simulink library "halout"  (R2021b)
settings: Solver=VariableStepAuto  StartTime=0.0  StopTime=10.0  RelTol=1e-3
undefined symbols (not defined in the file): C_TASK_5MS_S, FALSE, KHAL_CAN1TxReq_flg, KHAL_CAN2TxReq_flg, KHAL_CAN3FD3VCU1toNIDECTxReq_flg, KHAL_CAN3FD3VCU1TxReq_flg, KHAL_CAN3FD3VCU2E2E_flg, KHAL_CAN3FD3VCU2toNIDECE2E_flg, KHAL_CAN3FD3VCU2toNIDECTxReq_flg, KHAL_CAN3FD3VCU2TxReq_flg, KHAL_CAN3TxReq_flg, KHAL_CAN4FD4CE1000E2E_flg, KHAL_CAN4FD4CE1000TxReq_flg, KHAL_CAN4TxReq_flg, KHAL_CAN5TxReq_flg, KHAL_CAN7TxReq_flg, ONE_INT, TRUE, ZERO_INT
libraries: FVT_lib x258, simulink x115
(part 11 of 17)

== system halout/HAL_OUT/CAN2/FD2_CE200_1_0x435/FDCBCMKey2AccSta ==
  FDCBCMKey2AccSta : Inport
  Data Type Conversion : DataTypeConversion  OutDataTypeStr=uint8  RndMeth=Round
  CAN2_FDC_BCM_Key2Acc_Sta : Outport
  wires:
  Data Type Conversion/1 -> CAN2_FDC_BCM_Key2Acc_Sta/1
  FDCBCMKey2AccSta/1 -> Data Type Conversion/1

== system halout/HAL_OUT/CAN2/FD2_CE200_1_0x435/FDCBCMKey3AccSta ==
  FDCBCMKey3AccSta : Inport
  Data Type Conversion : DataTypeConversion  OutDataTypeStr=uint8  RndMeth=Round
  CAN2_FDC_BCM_Key3Acc_Sta : Outport
  wires:
  Data Type Conversion/1 -> CAN2_FDC_BCM_Key3Acc_Sta/1
  FDCBCMKey3AccSta/1 -> Data Type Conversion/1

== system halout/HAL_OUT/CAN2/FD2_CE200_1_0x435/FDCBCMKey4AccSta ==
  FDCBCMKey4AccSta : Inport
  Data Type Conversion : DataTypeConversion  OutDataTypeStr=uint8  RndMeth=Round
  CAN2_FDC_BCM_Key4Acc_Sta : Outport
  wires:
  Data Type Conversion/1 -> CAN2_FDC_BCM_Key4Acc_Sta/1
  FDCBCMKey4AccSta/1 -> Data Type Conversion/1

== system halout/HAL_OUT/CAN2/FD2_CE200_1_0x435/FDCBCMKey5AccSta ==
  FDCBCMKey5AccSta : Inport
  Data Type Conversion : DataTypeConversion  OutDataTypeStr=uint8  RndMeth=Round
  CAN2_FDC_BCM_Key5Acc_Sta : Outport
  wires:
  Data Type Conversion/1 -> CAN2_FDC_BCM_Key5Acc_Sta/1
  FDCBCMKey5AccSta/1 -> Data Type Conversion/1

== system halout/HAL_OUT/CAN2/FD2_CE200_1_0x435/FDCBCMKey6AccSta ==
  FDCBCMKey6AccSta : Inport
  Data Type Conversion : DataTypeConversion  OutDataTypeStr=uint8  RndMeth=Round
  CAN2_FDC_BCM_Key6Acc_Sta : Outport
  wires:
  Data Type Conversion/1 -> CAN2_FDC_BCM_Key6Acc_Sta/1
  FDCBCMKey6AccSta/1 -> Data Type Conversion/1

== system halout/HAL_OUT/CAN2/FD2_CE200_1_0x435/FDCBCMKey7AccSta ==
  FDCBCMKey7AccSta : Inport
  Data Type Conversion : DataTypeConversion  OutDataTypeStr=uint8  RndMeth=Round
  CAN2_FDC_BCM_Key7Acc_Sta : Outport
  wires:
  Data Type Conversion/1 -> CAN2_FDC_BCM_Key7Acc_Sta/1
  FDCBCMKey7AccSta/1 -> Data Type Conversion/1

== system halout/HAL_OUT/CAN2/FD2_CE200_1_0x435/FDCBCMKey8AccSta ==
  FDCBCMKey8AccSta : Inport
  Data Type Conversion : DataTypeConversion  OutDataTypeStr=uint8  RndMeth=Round
  CAN2_FDC_BCM_Key8Acc_Sta : Outport
  wires:
  Data Type Conversion/1 -> CAN2_FDC_BCM_Key8Acc_Sta/1
  FDCBCMKey8AccSta/1 -> Data Type Conversion/1

== system halout/HAL_OUT/CAN2/FD2_CE200_1_0x435/FDCBCMKey9AccSta ==
  FDCBCMKey9AccSta : Inport
  Data Type Conversion : DataTypeConversion  OutDataTypeStr=uint8  RndMeth=Round
  CAN2_FDC_BCM_Key9Acc_Sta : Outport
  wires:
  Data Type Conversion/1 -> CAN2_FDC_BCM_Key9Acc_Sta/1
  FDCBCMKey9AccSta/1 -> Data Type Conversion/1

== system halout/HAL_OUT/CAN2/FD2_CE200_1_0x435/FDCBCMLockAlarmCmd ==
  FDCBCMLockAlarmCmd : Inport
  Data Type Conversion : DataTypeConversion  OutDataTypeStr=uint8  RndMeth=Round
  CAN2_FDC_BCM_LockAlarm_Cmd : Outport
  wires:
  Data Type Conversion/1 -> CAN2_FDC_BCM_LockAlarm_Cmd/1
  FDCBCMLockAlarmCmd/1 -> Data Type Conversion/1

== system halout/HAL_OUT/CAN2/FD2_CE200_1_0x435/FDCBCMPTGOpenHeightSta ==
  FDCBCMPTGOpenHeightSta : Inport
  Data Type Conversion : DataTypeConversion  OutDataTypeStr=uint8  RndMeth=Round
  CAN2_FDC_BCM_PTGOpenHeight_Sta : Outport
  wires:
  Data Type Conversion/1 -> CAN2_FDC_BCM_PTGOpenHeight_Sta/1
  FDCBCMPTGOpenHeightSta/1 -> Data Type Conversion/1

== system halout/HAL_OUT/CAN2/FD2_CE200_1_0x435/FDCBCMRmLpModeENFunSta ==
  FDCBCMRmLpModeENFunSta : Inport
  Data Type Conversion : DataTypeConversion  OutDataTypeStr=uint8  RndMeth=Round
  CAN2_FDC_BCM_RmLpModeENFun_Sta : Outport
  wires:
  Data Type Conversion/1 -> CAN2_FDC_BCM_RmLpModeENFun_Sta/1
  FDCBCMRmLpModeENFunSta/1 -> Data Type Conversion/1

== system halout/HAL_OUT/CAN2/FD2_CE200_1_0x435/FDCBCMTurnSwTSetStaSta ==
  FDCBCMTurnSwTSetStaSta : Inport
  Data Type Conversion : DataTypeConversion  OutDataTypeStr=uint8  RndMeth=Round
  CAN2_FDC_BCM_TurnSwTSetSta_Sta : Outport
  wires:
  Data Type Conversion/1 -> CAN2_FDC_BCM_TurnSwTSetSta_Sta/1
  FDCBCMTurnSwTSetStaSta/1 -> Data Type Conversion/1

== system halout/HAL_OUT/CAN2/FD2_CE200_1_0x435/FDCBCMUserNowSta ==
  FDCBCMUserNowSta : Inport
  Data Type Conversion : DataTypeConversion  OutDataTypeStr=uint8  RndMeth=Round
  CAN2_FDC_BCM_UserNow_Sta : Outport
  wires:
  Data Type Conversion/1 -> CAN2_FDC_BCM_UserNow_Sta/1
  FDCBCMUserNowSta/1 -> Data Type Conversion/1

== system halout/HAL_OUT/CAN2/FD2_CE200_1_0x435/FDCBCMWalkInUnLkEnFunSta ==
  FDCBCMWalkInUnLkEnFunSta : Inport
  Data Type Conversion : DataTypeConversion  OutDataTypeStr=uint8  RndMeth=Round
  CAN2_FDC_BCM_WalkInUnLkEnFun_Sta : Outport
  wires:
  Data Type Conversion/1 -> CAN2_FDC_BCM_WalkInUnLkEnFun_Sta/1
  FDCBCMWalkInUnLkEnFunSta/1 -> Data Type Conversion/1

== system halout/HAL_OUT/CAN2/FD2_CE200_1_0x435/FDCBCMWalkOutLkEnFunSta ==
  FDCBCMWalkOutLkEnFunSta : Inport
  Data Type Conversion : DataTypeConversion  OutDataTypeStr=uint8  RndMeth=Round
  CAN2_FDC_BCM_WalkOutLkEnFun_Sta : Outport
  wires:
  Data Type Conversion/1 -> CAN2_FDC_BCM_WalkOutLkEnFun_Sta/1
  FDCBCMWalkOutLkEnFunSta/1 -> Data Type Conversion/1

== system halout/HAL_OUT/CAN2/FD2_CE200_1_0x435/FDCDKCDkeyShowIVISta ==
  FDCDKCDkeyShowIVISta : Inport
  Data Type Conversion : DataTypeConversion  OutDataTypeStr=uint8  RndMeth=Round
  CAN2_FDC_DKC_DkeyShowIVI_Sta : Outport
  wires:
  Data Type Conversion/1 -> CAN2_FDC_DKC_DkeyShowIVI_Sta/1
  FDCDKCDkeyShowIVISta/1 -> Data Type Conversion/1

== system halout/HAL_OUT/CAN2/FD2_CE200_1_0x435/FDCDKCKeyMissSta ==
  FDCDKCKeyMissSta : Inport
  Data Type Conversion : DataTypeConversion  OutDataTypeStr=uint8  RndMeth=Round
  CAN2_FDC_DKC_KeyMiss_Sta : Outport
  wires:
  Data Type Conversion/1 -> CAN2_FDC_DKC_KeyMiss_Sta/1
  FDCDKCKeyMissSta/1 -> Data Type Conversion/1

== system halout/HAL_OUT/CAN2/FD2_CE200_1_0x435/FDCDKCKeyNumSta ==
  FDCDKCKeyNumSta : Inport
  Data Type Conversion : DataTypeConversion  OutDataTypeStr=uint8  RndMeth=Round
  CAN2_FDC_DKC_KeyNum_Sta : Outport
  wires:
  Data Type Conversion/1 -> CAN2_FDC_DKC_KeyNum_Sta/1
  FDCDKCKeyNumSta/1 -> Data Type Conversion/1

== system halout/HAL_OUT/CAN2/FD2_CE200_1_0x435/FDCDKCKeyTypeSta ==
  FDCDKCKeyTypeSta : Inport
  Data Type Conversion : DataTypeConversion  OutDataTypeStr=uint8  RndMeth=Round
  CAN2_FDC_DKC_KeyType_Sta : Outport
  wires:
  Data Type Conversion/1 -> CAN2_FDC_DKC_KeyType_Sta/1
  FDCDKCKeyTypeSta/1 -> Data Type Conversion/1

== system halout/HAL_OUT/CAN2/FD2_CE200_1_0x435/FDCDKCUIDLowPowerSta ==
  FDCDKCUIDLowPowerSta : Inport
  Data Type Conversion : DataTypeConversion  OutDataTypeStr=uint8  RndMeth=Round
  CAN2_FDC_DKC_UIDLowPower_Sta : Outport
  wires:
  Data Type Conversion/1 -> CAN2_FDC_DKC_UIDLowPower_Sta/1
  FDCDKCUIDLowPowerSta/1 -> Data Type Conversion/1

== system halout/HAL_OUT/CAN2/FD2_CE200_1_0x435/FDCSPTGSPTGENFunSta ==
  FDCSPTGSPTGENFunSta : Inport
  Data Type Conversion : DataTypeConversion  OutDataTypeStr=uint8  RndMeth=Round
  CAN2_FDC_SPTG_SPTGENFun_Sta : Outport
  wires:
  Data Type Conversion/1 -> CAN2_FDC_SPTG_SPTGENFun_Sta/1
  FDCSPTGSPTGENFunSta/1 -> Data Type Conversion/1

== system halout/HAL_OUT/CAN2/FD2_CE200_1_0x435/FDCTHCMAPTCForceOFFSta ==
  FDCTHCMAPTCForceOFFSta : Inport
  Data Type Conversion : DataTypeConversion  OutDataTypeStr=uint8  RndMeth=Round
  CAN2_FDC_THCM_APTCForceOFF_Sta : Outport
  wires:
  Data Type Conversion/1 -> CAN2_FDC_THCM_APTCForceOFF_Sta/1
  FDCTHCMAPTCForceOFFSta/1 -> Data Type Conversion/1

== system halout/HAL_OUT/CAN2/FD2_CE200_1_0x435/FDCTHCMAPTCWarningSta ==
  FDCTHCMAPTCWarningSta : Inport
  Data Type Conversion : DataTypeConversion  OutDataTypeStr=uint8  RndMeth=Round
  CAN2_FDC_THCM_APTCWarning_Sta : Outport
  wires:
  Data Type Conversion/1 -> CAN2_FDC_THCM_APTCWarning_Sta/1
  FDCTHCMAPTCWarningSta/1 -> Data Type Conversion/1

== system halout/HAL_OUT/CAN2/FD2_CE200_1_0x435/FDCTHCMAirIntZ3Sta ==
  FDCTHCMAirIntZ3Sta : Inport
  Data Type Conversion : DataTypeConversion  OutDataTypeStr=uint8  RndMeth=Round
  CAN2_FDC_THCM_AirIntZ3_Sta : Outport
  wires:
  Data Type Conversion/1 -> CAN2_FDC_THCM_AirIntZ3_Sta/1
  FDCTHCMAirIntZ3Sta/1 -> Data Type Conversion/1

== system halout/HAL_OUT/CAN2/FD2_CE200_1_0x435/LFWheelShield ==
  LFWheelShield : Inport
  Data Type Conversion : DataTypeConversion  OutDataTypeStr=uint8  RndMeth=Round
  CAN2_LFWheelShield : Outport
  wires:
  Data Type Conversion/1 -> CAN2_LFWheelShield/1
  LFWheelShield/1 -> Data Type Conversion/1

== system halout/HAL_OUT/CAN2/FD2_CE200_1_0x435/LRBatWarn ==
  LRBatWarn : Inport
  Data Type Conversion : DataTypeConversion  OutDataTypeStr=uint8  RndMeth=Round
  CAN2_LRBatWarn : Outport
  wires:
  Data Type Conversion/1 -> CAN2_LRBatWarn/1
  LRBatWarn/1 -> Data Type Conversion/1

== system halout/HAL_OUT/CAN2/FD2_CE200_1_0x435/LRPressIndi ==
  LRPressIndi : Inport
  Data Type Conversion : DataTypeConversion  OutDataTypeStr=uint8  RndMeth=Round
  CAN2_LRPressIndi : Outport
  wires:
  Data Type Conversion/1 -> CAN2_LRPressIndi/1
  LRPressIndi/1 -> Data Type Conversion/1

== system halout/HAL_OUT/CAN2/FD2_CE200_1_0x435/LRSensorFail ==
  LRSensorFail : Inport
  Data Type Conversion : DataTypeConversion  OutDataTypeStr=uint8  RndMeth=Round
  CAN2_LRSensorFail : Outport
  wires:
  Data Type Conversion/1 -> CAN2_LRSensorFail/1
  LRSensorFail/1 -> Data Type Conversion/1

== system halout/HAL_OUT/CAN2/FD2_CE200_1_0x435/LRWheelDebug ==
  LRWheelDebug : Inport
  Data Type Conversion : DataTypeConversion  OutDataTypeStr=uint8  RndMeth=Round
  CAN2_LRWheelDebug : Outport
  wires:
  Data Type Conversion/1 -> CAN2_LRWheelDebug/1
  LRWheelDebug/1 -> Data Type Conversion/1

== system halout/HAL_OUT/CAN2/FD2_CE200_1_0x435/LRWheelPSW ==
  LRWheelPSW : Inport
  Data Type Conversion : DataTypeConversion  OutDataTypeStr=uint8  RndMeth=Round
  CAN2_LRWheelPSW : Outport
  wires:
  Data Type Conversion/1 -> CAN2_LRWheelPSW/1
  LRWheelPSW/1 -> Data Type Conversion/1

== system halout/HAL_OUT/CAN2/FD2_CE200_1_0x435/LRWheelPress ==
  LRWheelPress : Inport
  Data Type Conversion : DataTypeConversion  OutDataTypeStr=uint8  RndMeth=Round
  CAN2_LRWheelPress : Outport
  wires:
  Data Type Conversion/1 -> CAN2_LRWheelPress/1
  LRWheelPress/1 -> Data Type Conversion/1

== system halout/HAL_OUT/CAN2/FD2_CE200_1_0x435/LRWheelShield ==
  LRWheelShield : Inport
  Data Type Conversion : DataTypeConversion  OutDataTypeStr=uint8  RndMeth=Round
  CAN2_LRWheelShield : Outport
  wires:
  Data Type Conversion/1 -> CAN2_LRWheelShield/1
  LRWheelShield/1 -> Data Type Conversion/1

== system halout/HAL_OUT/CAN2/FD2_CE200_1_0x435/LRWheelTemp ==
  LRWheelTemp : Inport
  Data Type Conversion : DataTypeConversion  OutDataTypeStr=uint8  RndMeth=Round
  convert_out : FVT_lib/hal/convert_out  gain=1  offset=-40
  CAN2_LRWheelTemp : Outport
  wires:
  Data Type Conversion/1 -> CAN2_LRWheelTemp/1
  convert_out/1 -> Data Type Conversion/1
  LRWheelTemp/1 -> convert_out/1

== system halout/HAL_OUT/CAN2/FD2_CE200_1_0x435/LRWheelTmpIndi ==
  LRWheelTmpIndi : Inport
  Data Type Conversion : DataTypeConversion  OutDataTypeStr=uint8  RndMeth=Round
  CAN2_LRWheelTmpIndi : Outport
  wires:
  Data Type Conversion/1 -> CAN2_LRWheelTmpIndi/1
  LRWheelTmpIndi/1 -> Data Type Conversion/1

== system halout/HAL_OUT/CAN2/FD2_CE200_1_0x435/RFWheelShield ==
  RFWheelShield : Inport
  Data Type Conversion : DataTypeConversion  OutDataTypeStr=uint8  RndMeth=Round
  CAN2_RFWheelShield : Outport
  wires:
  Data Type Conversion/1 -> CAN2_RFWheelShield/1
  RFWheelShield/1 -> Data Type Conversion/1

== system halout/HAL_OUT/CAN2/FD2_CE200_1_0x435/RRBatWarn ==
  RRBatWarn : Inport
  Data Type Conversion : DataTypeConversion  OutDataTypeStr=uint8  RndMeth=Round
  CAN2_RRBatWarn : Outport
  wires:
  Data Type Conversion/1 -> CAN2_RRBatWarn/1
  RRBatWarn/1 -> Data Type Conversion/1

== system halout/HAL_OUT/CAN2/FD2_CE200_1_0x435/RRPressIndi ==
  RRPressIndi : Inport
  Data Type Conversion : DataTypeConversion  OutDataTypeStr=uint8  RndMeth=Round
  CAN2_RRPressIndi : Outport
  wires:
  Data Type Conversion/1 -> CAN2_RRPressIndi/1
  RRPressIndi/1 -> Data Type Conversion/1

== system halout/HAL_OUT/CAN2/FD2_CE200_1_0x435/RRSensorFail ==
  RRSensorFail : Inport
  Data Type Conversion : DataTypeConversion  OutDataTypeStr=uint8  RndMeth=Round
  CAN2_RRSensorFail : Outport
  wires:
  Data Type Conversion/1 -> CAN2_RRSensorFail/1
  RRSensorFail/1 -> Data Type Conversion/1

== system halout/HAL_OUT/CAN2/FD2_CE200_1_0x435/RRWheelDebug ==
  RRWheelDebug : Inport
  Data Type Conversion : DataTypeConversion  OutDataTypeStr=uint8  RndMeth=Round
  CAN2_RRWheelDebug : Outport
  wires:
  Data Type Conversion/1 -> CAN2_RRWheelDebug/1
  RRWheelDebug/1 -> Data Type Conversion/1

== system halout/HAL_OUT/CAN2/FD2_CE200_1_0x435/RRWheelPSW ==
  RRWheelPSW : Inport
  Data Type Conversion : DataTypeConversion  OutDataTypeStr=uint8  RndMeth=Round
  CAN2_RRWheelPSW : Outport
  wires:
  Data Type Conversion/1 -> CAN2_RRWheelPSW/1
  RRWheelPSW/1 -> Data Type Conversion/1

== system halout/HAL_OUT/CAN2/FD2_CE200_1_0x435/RRWheelPress ==
  RRWheelPress : Inport
  Data Type Conversion : DataTypeConversion  OutDataTypeStr=uint8  RndMeth=Round
  CAN2_RRWheelPress : Outport
  wires:
  Data Type Conversion/1 -> CAN2_RRWheelPress/1
  RRWheelPress/1 -> Data Type Conversion/1

== system halout/HAL_OUT/CAN2/FD2_CE200_1_0x435/RRWheelShield ==
  RRWheelShield : Inport
  Data Type Conversion : DataTypeConversion  OutDataTypeStr=uint8  RndMeth=Round
  CAN2_RRWheelShield : Outport
  wires:
  Data Type Conversion/1 -> CAN2_RRWheelShield/1
  RRWheelShield/1 -> Data Type Conversion/1

== system halout/HAL_OUT/CAN2/FD2_CE200_1_0x435/RRWheelTemp ==
  RRWheelTemp : Inport
  Data Type Conversion : DataTypeConversion  OutDataTypeStr=uint8  RndMeth=Round
  convert_out : FVT_lib/hal/convert_out  gain=1  offset=-40
  CAN2_RRWheelTemp : Outport
  wires:
  Data Type Conversion/1 -> CAN2_RRWheelTemp/1
  convert_out/1 -> Data Type Conversion/1
  RRWheelTemp/1 -> convert_out/1

== system halout/HAL_OUT/CAN2/FD2_CE200_1_0x435/RRWheelTmpIndi ==
  RRWheelTmpIndi : Inport
  Data Type Conversion : DataTypeConversion  OutDataTypeStr=uint8  RndMeth=Round
  CAN2_RRWheelTmpIndi : Outport
  wires:
  Data Type Conversion/1 -> CAN2_RRWheelTmpIndi/1
  RRWheelTmpIndi/1 -> Data Type Conversion/1

== system halout/HAL_OUT/CAN2/FD2_CE200_1_0x435/T1TPMSLFBatWarn ==
  T1TPMSLFBatWarn : Inport
  Data Type Conversion : DataTypeConversion  OutDataTypeStr=uint8  RndMeth=Round
  CAN2_T1_TPMS_LFBatWarn : Outport
  wires:
  Data Type Conversion/1 -> CAN2_T1_TPMS_LFBatWarn/1
  T1TPMSLFBatWarn/1 -> Data Type Conversion/1

== system halout/HAL_OUT/CAN2/FD2_CE200_1_0x435/T1TPMSLFPressIndi ==
  T1TPMSLFPressIndi : Inport
  Data Type Conversion : DataTypeConversion  OutDataTypeStr=uint8  RndMeth=Round
  CAN2_T1_TPMS_LFPressIndi : Outport
  wires:
  Data Type Conversion/1 -> CAN2_T1_TPMS_LFPressIndi/1
  T1TPMSLFPressIndi/1 -> Data Type Conversion/1

== system halout/HAL_OUT/CAN2/FD2_CE200_1_0x435/T1TPMSLFSensorFail ==
  T1TPMSLFSensorFail : Inport
  Data Type Conversion : DataTypeConversion  OutDataTypeStr=uint8  RndMeth=Round
  CAN2_T1_TPMS_LFSensorFail : Outport
  wires:
  Data Type Conversion/1 -> CAN2_T1_TPMS_LFSensorFail/1
  T1TPMSLFSensorFail/1 -> Data Type Conversion/1

== system halout/HAL_OUT/CAN2/FD2_CE200_1_0x435/T1TPMSLFWheelDebug ==
  T1TPMSLFWheelDebug : Inport
  Data Type Conversion : DataTypeConversion  OutDataTypeStr=uint8  RndMeth=Round
  CAN2_T1_TPMS_LFWheelDebug : Outport
  wires:
  Data Type Conversion/1 -> CAN2_T1_TPMS_LFWheelDebug/1
  T1TPMSLFWheelDebug/1 -> Data Type Conversion/1

== system halout/HAL_OUT/CAN2/FD2_CE200_1_0x435/T1TPMSLFWheelPSW ==
  T1TPMSLFWheelPSW : Inport
  Data Type Conversion : DataTypeConversion  OutDataTypeStr=uint8  RndMeth=Round
  CAN2_T1_TPMS_LFWheelPSW : Outport
  wires:
  Data Type Conversion/1 -> CAN2_T1_TPMS_LFWheelPSW/1
  T1TPMSLFWheelPSW/1 -> Data Type Conversion/1

== system halout/HAL_OUT/CAN2/FD2_CE200_1_0x435/T1TPMSLFWheelPress ==
  T1TPMSLFWheelPress : Inport
  Data Type Conversion : DataTypeConversion  OutDataTypeStr=uint8  RndMeth=Round
  CAN2_T1_TPMS_LFWheelPress : Outport
  wires:
  Data Type Conversion/1 -> CAN2_T1_TPMS_LFWheelPress/1
  T1TPMSLFWheelPress/1 -> Data Type Conversion/1

== system halout/HAL_OUT/CAN2/FD2_CE200_1_0x435/T1TPMSLFWheelTemp ==
  T1TPMSLFWheelTemp : Inport
  Data Type Conversion : DataTypeConversion  OutDataTypeStr=uint8  RndMeth=Round
  convert_out : FVT_lib/hal/convert_out  gain=1  offset=-40
  CAN2_T1_TPMS_LFWheelTemp : Outport
  wires:
  Data Type Conversion/1 -> CAN2_T1_TPMS_LFWheelTemp/1
  convert_out/1 -> Data Type Conversion/1
  T1TPMSLFWheelTemp/1 -> convert_out/1

== system halout/HAL_OUT/CAN2/FD2_CE200_1_0x435/T1TPMSLFWheelTmpIndi ==
  T1TPMSLFWheelTmpIndi : Inport
  Data Type Conversion : DataTypeConversion  OutDataTypeStr=uint8  RndMeth=Round
  CAN2_T1_TPMS_LFWheelTmpIndi : Outport
  wires:
  Data Type Conversion/1 -> CAN2_T1_TPMS_LFWheelTmpIndi/1
  T1TPMSLFWheelTmpIndi/1 -> Data Type Conversion/1

== system halout/HAL_OUT/CAN2/FD2_CE200_1_0x435/T1TPMSRFBatWarn ==
  T1TPMSRFBatWarn : Inport
  Data Type Conversion : DataTypeConversion  OutDataTypeStr=uint8  RndMeth=Round
  CAN2_T1_TPMS_RFBatWarn : Outport
  wires:
  Data Type Conversion/1 -> CAN2_T1_TPMS_RFBatWarn/1
  T1TPMSRFBatWarn/1 -> Data Type Conversion/1

== system halout/HAL_OUT/CAN2/FD2_CE200_1_0x435/T1TPMSRFPressIndi ==
  T1TPMSRFPressIndi : Inport
  Data Type Conversion : DataTypeConversion  OutDataTypeStr=uint8  RndMeth=Round
  CAN2_T1_TPMS_RFPressIndi : Outport
  wires:
  Data Type Conversion/1 -> CAN2_T1_TPMS_RFPressIndi/1
  T1TPMSRFPressIndi/1 -> Data Type Conversion/1

== system halout/HAL_OUT/CAN2/FD2_CE200_1_0x435/T1TPMSRFSensorFail ==
  T1TPMSRFSensorFail : Inport
  Data Type Conversion : DataTypeConversion  OutDataTypeStr=uint8  RndMeth=Round
  CAN2_T1_TPMS_RFSensorFail : Outport
  wires:
  Data Type Conversion/1 -> CAN2_T1_TPMS_RFSensorFail/1
  T1TPMSRFSensorFail/1 -> Data Type Conversion/1

== system halout/HAL_OUT/CAN2/FD2_CE200_1_0x435/T1TPMSRFWheelDebug ==
  T1TPMSRFWheelDebug : Inport
  Data Type Conversion : DataTypeConversion  OutDataTypeStr=uint8  RndMeth=Round
  CAN2_T1_TPMS_RFWheelDebug : Outport
  wires:
  Data Type Conversion/1 -> CAN2_T1_TPMS_RFWheelDebug/1
  T1TPMSRFWheelDebug/1 -> Data Type Conversion/1

== system halout/HAL_OUT/CAN2/FD2_CE200_1_0x435/T1TPMSRFWheelPSW ==
  T1TPMSRFWheelPSW : Inport
  Data Type Conversion : DataTypeConversion  OutDataTypeStr=uint8  RndMeth=Round
  CAN2_T1_TPMS_RFWheelPSW : Outport
  wires:
  Data Type Conversion/1 -> CAN2_T1_TPMS_RFWheelPSW/1
  T1TPMSRFWheelPSW/1 -> Data Type Conversion/1

== system halout/HAL_OUT/CAN2/FD2_CE200_1_0x435/T1TPMSRFWheelPress ==
  T1TPMSRFWheelPress : Inport
  Data Type Conversion : DataTypeConversion  OutDataTypeStr=uint8  RndMeth=Round
  CAN2_T1_TPMS_RFWheelPress : Outport
  wires:
  Data Type Conversion/1 -> CAN2_T1_TPMS_RFWheelPress/1
  T1TPMSRFWheelPress/1 -> Data Type Conversion/1

== system halout/HAL_OUT/CAN2/FD2_CE200_1_0x435/T1TPMSRFWheelTemp ==
  T1TPMSRFWheelTemp : Inport
  Data Type Conversion : DataTypeConversion  OutDataTypeStr=uint8  RndMeth=Round
  convert_out : FVT_lib/hal/convert_out  gain=1  offset=-40
  CAN2_T1_TPMS_RFWheelTemp : Outport
  wires:
  Data Type Conversion/1 -> CAN2_T1_TPMS_RFWheelTemp/1
  convert_out/1 -> Data Type Conversion/1
  T1TPMSRFWheelTemp/1 -> convert_out/1

== system halout/HAL_OUT/CAN2/FD2_CE200_1_0x435/T1TPMSRFWheelTmpIndi ==
  T1TPMSRFWheelTmpIndi : Inport
  Data Type Conversion : DataTypeConversion  OutDataTypeStr=uint8  RndMeth=Round
  CAN2_T1_TPMS_RFWheelTmpIndi : Outport
  wires:
  Data Type Conversion/1 -> CAN2_T1_TPMS_RFWheelTmpIndi/1
  T1TPMSRFWheelTmpIndi/1 -> Data Type Conversion/1

== system halout/HAL_OUT/CAN2/FD2_CE200_1_0x435/T1TPMSTPMSWarnIndi ==
  T1TPMSTPMSWarnIndi : Inport
  Data Type Conversion : DataTypeConversion  OutDataTypeStr=uint8  RndMeth=Round
  CAN2_T1_TPMS_TPMSWarnIndi : Outport
  wires:
  Data Type Conversion/1 -> CAN2_T1_TPMS_TPMSWarnIndi/1
  T1TPMSTPMSWarnIndi/1 -> Data Type Conversion/1

== system halout/HAL_OUT/CAN2/FD2_CE200_1_0x435/TPMSCaliButtAllow ==
  TPMSCaliButtAllow : Inport
  Data Type Conversion : DataTypeConversion  OutDataTypeStr=uint8  RndMeth=Round
  CAN2_TPMS_Cali_Butt_Allow : Outport
  wires:
  Data Type Conversion/1 -> CAN2_TPMS_Cali_Butt_Allow/1
  TPMSCaliButtAllow/1 -> Data Type Conversion/1

== system halout/HAL_OUT/CAN2/FD2_CE200_1_0x435/TPMSResButtAllow ==
  TPMSResButtAllow : Inport
  Data Type Conversion : DataTypeConversion  OutDataTypeStr=uint8  RndMeth=Round
  CAN2_TPMS_Res_Butt_Allow : Outport
  wires:
  Data Type Conversion/1 -> CAN2_TPMS_Res_Butt_Allow/1
  TPMSResButtAllow/1 -> Data Type Conversion/1

== system halout/HAL_OUT/CAN2/FD2_Version_0x3C3/FUSIONHWVer1 ==
  FUSIONHWVer1 : Inport
  Data Type Conversion : DataTypeConversion  OutDataTypeStr=uint8  RndMeth=Round
  CAN2_FUSION_HW_Ver1 : Outport
  wires:
  Data Type Conversion/1 -> CAN2_FUSION_HW_Ver1/1
  FUSIONHWVer1/1 -> Data Type Conversion/1

== system halout/HAL_OUT/CAN2/FD2_Version_0x3C3/FUSIONHWVer2 ==
  FUSIONHWVer2 : Inport
  Data Type Conversion : DataTypeConversion  OutDataTypeStr=uint8  RndMeth=Round
  CAN2_FUSION_HW_Ver2 : Outport
  wires:
  Data Type Conversion/1 -> CAN2_FUSION_HW_Ver2/1
  FUSIONHWVer2/1 -> Data Type Conversion/1

== system halout/HAL_OUT/CAN2/FD2_Version_0x3C3/FUSIONHWVer3 ==
  FUSIONHWVer3 : Inport
  Data Type Conversion : DataTypeConversion  OutDataTypeStr=uint8  RndMeth=Round
  CAN2_FUSION_HW_Ver3 : Outport
  wires:
  Data Type Conversion/1 -> CAN2_FUSION_HW_Ver3/1
  FUSIONHWVer3/1 -> Data Type Conversion/1

== system halout/HAL_OUT/CAN2/FD2_Version_0x3C3/FUSIONSWCarModel1 ==
  FUSIONSWCarModel1 : Inport
  Data Type Conversion : DataTypeConversion  OutDataTypeStr=uint8  RndMeth=Round
  CAN2_FUSION_SW_CarModel1 : Outport
  wires:
  Data Type Conversion/1 -> CAN2_FUSION_SW_CarModel1/1
  FUSIONSWCarModel1/1 -> Data Type Conversion/1

== system halout/HAL_OUT/CAN2/FD2_Version_0x3C3/FUSIONSWCarModel2 ==
  FUSIONSWCarModel2 : Inport
  Data Type Conversion : DataTypeConversion  OutDataTypeStr=uint8  RndMeth=Round
  CAN2_FUSION_SW_CarModel2 : Outport
  wires:
  Data Type Conversion/1 -> CAN2_FUSION_SW_CarModel2/1
  FUSIONSWCarModel2/1 -> Data Type Conversion/1

== system halout/HAL_OUT/CAN2/FD2_Version_0x3C3/FUSIONSWCarModel3 ==
  FUSIONSWCarModel3 : Inport
  Data Type Conversion : DataTypeConversion  OutDataTypeStr=uint8  RndMeth=Round
  CAN2_FUSION_SW_CarModel3 : Outport
  wires:
  Data Type Conversion/1 -> CAN2_FUSION_SW_CarModel3/1
  FUSIONSWCarModel3/1 -> Data Type Conversion/1

== system halout/HAL_OUT/CAN2/FD2_Version_0x3C3/FUSIONSWController1 ==
  FUSIONSWController1 : Inport
  Data Type Conversion : DataTypeConversion  OutDataTypeStr=uint8  RndMeth=Round
  CAN2_FUSION_SW_Controller1 : Outport
  wires:
  Data Type Conversion/1 -> CAN2_FUSION_SW_Controller1/1
  FUSIONSWController1/1 -> Data Type Conversion/1

== system halout/HAL_OUT/CAN2/FD2_Version_0x3C3/FUSIONSWController2 ==
  FUSIONSWController2 : Inport
  Data Type Conversion : DataTypeConversion  OutDataTypeStr=uint8  RndMeth=Round
  CAN2_FUSION_SW_Controller2 : Outport
  wires:
  Data Type Conversion/1 -> CAN2_FUSION_SW_Controller2/1
  FUSIONSWController2/1 -> Data Type Conversion/1

== system halout/HAL_OUT/CAN2/FD2_Version_0x3C3/FUSIONSWCountry1 ==
  FUSIONSWCountry1 : Inport
  Data Type Conversion : DataTypeConversion  OutDataTypeStr=uint8  RndMeth=Round
  CAN2_FUSION_SW_Country1 : Outport
  wires:
  Data Type Conversion/1 -> CAN2_FUSION_SW_Country1/1
  FUSIONSWCountry1/1 -> Data Type Conversion/1

== system halout/HAL_OUT/CAN2/FD2_Version_0x3C3/FUSIONSWCountry2 ==
  FUSIONSWCountry2 : Inport
  Data Type Conversion : DataTypeConversion  OutDataTypeStr=uint8  RndMeth=Round
  CAN2_FUSION_SW_Country2 : Outport
  wires:
  Data Type Conversion/1 -> CAN2_FUSION_SW_Country2/1
  FUSIONSWCountry2/1 -> Data Type Conversion/1

== system halout/HAL_OUT/CAN2/FD2_Version_0x3C3/FUSIONSWECUGen1 ==
  FUSIONSWECUGen1 : Inport
  Data Type Conversion : DataTypeConversion  OutDataTypeStr=uint8  RndMeth=Round
  CAN2_FUSION_SW_ECUGen1 : Outport
  wires:
  Data Type Conversion/1 -> CAN2_FUSION_SW_ECUGen1/1
  FUSIONSWECUGen1/1 -> Data Type Conversion/1

== system halout/HAL_OUT/CAN2/FD2_Version_0x3C3/FUSIONSWECUGen2 ==
  FUSIONSWECUGen2 : Inport
  Data Type Conversion : DataTypeConversion  OutDataTypeStr=uint8  RndMeth=Round
  CAN2_FUSION_SW_ECUGen2 : Outport
  wires:
  Data Type Conversion/1 -> CAN2_FUSION_SW_ECUGen2/1
  FUSIONSWECUGen2/1 -> Data Type Conversion/1

== system halout/HAL_OUT/CAN2/FD2_Version_0x3C3/FUSIONSWMajor1 ==
  FUSIONSWMajor1 : Inport
  Data Type Conversion : DataTypeConversion  OutDataTypeStr=uint8  RndMeth=Round
  CAN2_FUSION_SW_Major1 : Outport
  wires:
  Data Type Conversion/1 -> CAN2_FUSION_SW_Major1/1
  FUSIONSWMajor1/1 -> Data Type Conversion/1

== system halout/HAL_OUT/CAN2/FD2_Version_0x3C3/FUSIONSWMajor2 ==
  FUSIONSWMajor2 : Inport
  Data Type Conversion : DataTypeConversion  OutDataTypeStr=uint8  RndMeth=Round
  CAN2_FUSION_SW_Major2 : Outport
  wires:
  Data Type Conversion/1 -> CAN2_FUSION_SW_Major2/1
  FUSIONSWMajor2/1 -> Data Type Conversion/1

== system halout/HAL_OUT/CAN2/FD2_Version_0x3C3/FUSIONSWMinor1 ==
  FUSIONSWMinor1 : Inport
  Data Type Conversion : DataTypeConversion  OutDataTypeStr=uint8  RndMeth=Round
  CAN2_FUSION_SW_Minor1 : Outport
  wires:
  Data Type Conversion/1 -> CAN2_FUSION_SW_Minor1/1
  FUSIONSWMinor1/1 -> Data Type Conversion/1

== system halout/HAL_OUT/CAN2/FD2_Version_0x3C3/FUSIONSWMinor2 ==
  FUSIONSWMinor2 : Inport
  Data Type Conversion : DataTypeConversion  OutDataTypeStr=uint8  RndMeth=Round
  CAN2_FUSION_SW_Minor2 : Outport
  wires:
  Data Type Conversion/1 -> CAN2_FUSION_SW_Minor2/1
  FUSIONSWMinor2/1 -> Data Type Conversion/1

== system halout/HAL_OUT/CAN2/FD2_Version_0x3C3/FUSIONSWPatch1 ==
  FUSIONSWPatch1 : Inport
  Data Type Conversion : DataTypeConversion  OutDataTypeStr=uint8  RndMeth=Round
  CAN2_FUSION_SW_Patch1 : Outport
  wires:
  Data Type Conversion/1 -> CAN2_FUSION_SW_Patch1/1
  FUSIONSWPatch1/1 -> Data Type Conversion/1

== system halout/HAL_OUT/CAN2/FD2_Version_0x3C3/FUSIONSWPatch2 ==
  FUSIONSWPatch2 : Inport
  Data Type Conversion : DataTypeConversion  OutDataTypeStr=uint8  RndMeth=Round
  CAN2_FUSION_SW_Patch2 : Outport
  wires:
  Data Type Conversion/1 -> CAN2_FUSION_SW_Patch2/1
  FUSIONSWPatch2/1 -> Data Type Conversion/1

== system halout/HAL_OUT/CAN2/FD2_Version_0x3C3/FUSIONSWSHA1 ==
  FUSIONSWSHA1 : Inport
  Data Type Conversion : DataTypeConversion  OutDataTypeStr=uint8  RndMeth=Round
  CAN2_FUSION_SW_SHA1 : Outport
  wires:
  Data Type Conversion/1 -> CAN2_FUSION_SW_SHA1/1
  FUSIONSWSHA1/1 -> Data Type Conversion/1

== system halout/HAL_OUT/CAN2/FD2_Version_0x3C3/FUSIONSWSHA2 ==
  FUSIONSWSHA2 : Inport
  Data Type Conversion : DataTypeConversion  OutDataTypeStr=uint8  RndMeth=Round
  CAN2_FUSION_SW_SHA2 : Outport
  wires:
  Data Type Conversion/1 -> CAN2_FUSION_SW_SHA2/1
  FUSIONSWSHA2/1 -> Data Type Conversion/1

== system halout/HAL_OUT/CAN2/FD2_Version_0x3C3/FUSIONSWSHA3 ==
  FUSIONSWSHA3 : Inport
  Data Type Conversion : DataTypeConversion  OutDataTypeStr=uint8  RndMeth=Round
  CAN2_FUSION_SW_SHA3 : Outport
  wires:
  Data Type Conversion/1 -> CAN2_FUSION_SW_SHA3/1
  FUSIONSWSHA3/1 -> Data Type Conversion/1

== system halout/HAL_OUT/CAN2/FD2_Version_0x3C3/FUSIONSWSHA4 ==
  FUSIONSWSHA4 : Inport
  Data Type Conversion : DataTypeConversion  OutDataTypeStr=uint8  RndMeth=Round
  CAN2_FUSION_SW_SHA4 : Outport
  wires:
  Data Type Conversion/1 -> CAN2_FUSION_SW_SHA4/1
  FUSIONSWSHA4/1 -> Data Type Conversion/1

== system halout/HAL_OUT/CAN2/FD2_Version_0x3C3/FUSIONSWSHA5 ==
  FUSIONSWSHA5 : Inport
  Data Type Conversion : DataTypeConversion  OutDataTypeStr=uint8  RndMeth=Round
  CAN2_FUSION_SW_SHA5 : Outport
  wires:
  Data Type Conversion/1 -> CAN2_FUSION_SW_SHA5/1
  FUSIONSWSHA5/1 -> Data Type Conversion/1

== system halout/HAL_OUT/CAN2/FD2_Version_0x3C3/FUSIONSWSHA6 ==
  FUSIONSWSHA6 : Inport
  Data Type Conversion : DataTypeConversion  OutDataTypeStr=uint8  RndMeth=Round
  CAN2_FUSION_SW_SHA6 : Outport
  wires:
  Data Type Conversion/1 -> CAN2_FUSION_SW_SHA6/1
  FUSIONSWSHA6/1 -> Data Type Conversion/1

== system halout/HAL_OUT/CAN2/FD2_Version_0x3C3/FUSIONSWSHA7 ==
  FUSIONSWSHA7 : Inport
  Data Type Conversion : DataTypeConversion  OutDataTypeStr=uint8  RndMeth=Round
  CAN2_FUSION_SW_SHA7 : Outport
  wires:
  Data Type Conversion/1 -> CAN2_FUSION_SW_SHA7/1
  FUSIONSWSHA7/1 -> Data Type Conversion/1

== system halout/HAL_OUT/CAN2/FD2_Version_0x3C3/FUSIONSWSHA8 ==
  FUSIONSWSHA8 : Inport
  Data Type Conversion : DataTypeConversion  OutDataTypeStr=uint8  RndMeth=Round
  CAN2_FUSION_SW_SHA8 : Outport
  wires:
  Data Type Conversion/1 -> CAN2_FUSION_SW_SHA8/1
  FUSIONSWSHA8/1 -> Data Type Conversion/1

== system halout/HAL_OUT/CAN2/FD2_Version_0x3C3/FUSIONSWVar1 ==
  FUSIONSWVar1 : Inport
  Data Type Conversion : DataTypeConversion  OutDataTypeStr=uint8  RndMeth=Round
  CAN2_FUSION_SW_Var1 : Outport
  wires:
  Data Type Conversion/1 -> CAN2_FUSION_SW_Var1/1
  FUSIONSWVar1/1 -> Data Type Conversion/1

== system halout/HAL_OUT/CAN2/FD2_Version_0x3C3/FUSIONSWVar2 ==
  FUSIONSWVar2 : Inport
  Data Type Conversion : DataTypeConversion  OutDataTypeStr=uint8  RndMeth=Round
  CAN2_FUSION_SW_Var2 : Outport
  wires:
  Data Type Conversion/1 -> CAN2_FUSION_SW_Var2/1
  FUSIONSWVar2/1 -> Data Type Conversion/1

== system halout/HAL_OUT/CAN2/FD2_Version_0x3C3/FUSIONSWVar3 ==
  FUSIONSWVar3 : Inport
  Data Type Conversion : DataTypeConversion  OutDataTypeStr=uint8  RndMeth=Round
  CAN2_FUSION_SW_Var3 : Outport
  wires:
  Data Type Conversion/1 -> CAN2_FUSION_SW_Var3/1
  FUSIONSWVar3/1 -> Data Type Conversion/1

== system halout/HAL_OUT/CAN2/FD2_Version_0x3C3/FUSIONSWVar4 ==
  FUSIONSWVar4 : Inport
  Data Type Conversion : DataTypeConversion  OutDataTypeStr=uint8  RndMeth=Round
  CAN2_FUSION_SW_Var4 : Outport
  wires:
  Data Type Conversion/1 -> CAN2_FUSION_SW_Var4/1
  FUSIONSWVar4/1 -> Data Type Conversion/1

== system halout/HAL_OUT/CAN2/FD2_Version_0x3C3/FUSIONSWVar5 ==
  FUSIONSWVar5 : Inport
  Data Type Conversion : DataTypeConversion  OutDataTypeStr=uint8  RndMeth=Round
  CAN2_FUSION_SW_Var5 : Outport
  wires:
  Data Type Conversion/1 -> CAN2_FUSION_SW_Var5/1
  FUSIONSWVar5/1 -> Data Type Conversion/1

== system halout/HAL_OUT/CAN2/FD2_Version_0x3C3/FUSIONSWchange1 ==
  FUSIONSWchange1 : Inport
  Data Type Conversion : DataTypeConversion  OutDataTypeStr=uint8  RndMeth=Round
  CAN2_FUSION_SW_change1 : Outport
  wires:
  Data Type Conversion/1 -> CAN2_FUSION_SW_change1/1
  FUSIONSWchange1/1 -> Data Type Conversion/1

== system halout/HAL_OUT/CAN2/FD2_Version_0x3C3/FUSIONSWchange2 ==
  FUSIONSWchange2 : Inport
  Data Type Conversion : DataTypeConversion  OutDataTypeStr=uint8  RndMeth=Round
  CAN2_FUSION_SW_change2 : Outport
  wires:
  Data Type Conversion/1 -> CAN2_FUSION_SW_change2/1
  FUSIONSWchange2/1 -> Data Type Conversion/1

== system halout/HAL_OUT/CAN2/FD2_Version_0x3C3/FUSIONSWdash1 ==
  FUSIONSWdash1 : Inport
  Data Type Conversion : DataTypeConversion  OutDataTypeStr=uint8  RndMeth=Round
  CAN2_FUSION_SW_dash1 : Outport
  wires:
  Data Type Conversion/1 -> CAN2_FUSION_SW_dash1/1
  FUSIONSWdash1/1 -> Data Type Conversion/1

== system halout/HAL_OUT/CAN2/FD2_Version_0x3C3/FUSIONSWdash2 ==
  FUSIONSWdash2 : Inport
  Data Type Conversion : DataTypeConversion  OutDataTypeStr=uint8  RndMeth=Round
  CAN2_FUSION_SW_dash2 : Outport
  wires:
  Data Type Conversion/1 -> CAN2_FUSION_SW_dash2/1
  FUSIONSWdash2/1 -> Data Type Conversion/1

== system halout/HAL_OUT/CAN2/GW2_C10_0_0x1B3/ABSActive ==
  ABSActive : Inport
  Data Type Conversion : DataTypeConversion  OutDataTypeStr=uint8  RndMeth=Round
  CAN2_ABS_Active : Outport
  wires:
  Data Type Conversion/1 -> CAN2_ABS_Active/1
  ABSActive/1 -> Data Type Conversion/1

== system halout/HAL_OUT/CAN2/GW2_C10_0_0x1B3/ABSFailed ==
  ABSFailed : Inport
  Data Type Conversion : DataTypeConversion  OutDataTypeStr=uint8  RndMeth=Round
  CAN2_ABS_Failed : Outport
  wires:
  Data Type Conversion/1 -> CAN2_ABS_Failed/1
  ABSFailed/1 -> Data Type Conversion/1

== system halout/HAL_OUT/CAN2/GW2_C10_0_0x1B3/ABSWnlmpSta ==
  ABSWnlmpSta : Inport
  Data Type Conversion : DataTypeConversion  OutDataTypeStr=uint8  RndMeth=Round
  CAN2_ABS_WnlmpSta : Outport
  wires:
  Data Type Conversion/1 -> CAN2_ABS_WnlmpSta/1
  ABSWnlmpSta/1 -> Data Type Conversion/1

== system halout/HAL_OUT/CAN2/GW2_C10_0_0x1B3/AVHFailed ==
  AVHFailed : Inport
  Data Type Conversion : DataTypeConversion  OutDataTypeStr=uint8  RndMeth=Round
  CAN2_AVH_Failed : Outport
  wires:
  Data Type Conversion/1 -> CAN2_AVH_Failed/1
  AVHFailed/1 -> Data Type Conversion/1

== system halout/HAL_OUT/CAN2/GW2_C10_0_0x1B3/AmberWnlmpSta ==
  AmberWnlmpSta : Inport
  Data Type Conversion : DataTypeConversion  OutDataTypeStr=uint8  RndMeth=Round
  CAN2_Amber_WnlmpSta : Outport
  wires:
  Data Type Conversion/1 -> CAN2_Amber_WnlmpSta/1
  AmberWnlmpSta/1 -> Data Type Conversion/1

== system halout/HAL_OUT/CAN2/GW2_C10_0_0x1B3/BrkSwSta ==
  BrkSwSta : Inport
  Data Type Conversion : DataTypeConversion  OutDataTypeStr=uint8  RndMeth=Round
  CAN2_BrkSw_Sta : Outport
  wires:
  Data Type Conversion/1 -> CAN2_BrkSw_Sta/1
  BrkSwSta/1 -> Data Type Conversion/1

== system halout/HAL_OUT/CAN2/GW2_C10_0_0x1B3/HSAActive ==
  HSAActive : Inport
  Data Type Conversion : DataTypeConversion  OutDataTypeStr=uint8  RndMeth=Round
  CAN2_HSA_Active : Outport
  wires:
  Data Type Conversion/1 -> CAN2_HSA_Active/1
  HSAActive/1 -> Data Type Conversion/1

== system halout/HAL_OUT/CAN2/GW2_C10_0_0x1B3/HSAFailed ==
  HSAFailed : Inport
  Data Type Conversion : DataTypeConversion  OutDataTypeStr=uint8  RndMeth=Round
  CAN2_HSA_Failed : Outport
  wires:
  Data Type Conversion/1 -> CAN2_HSA_Failed/1
  HSAFailed/1 -> Data Type Conversion/1

== system halout/HAL_OUT/CAN2/GW2_C10_0_0x1B3/MeterIndVehSpeed ==
  MeterIndVehSpeed : Inport
  Data Type Conversion : DataTypeConversion  OutDataTypeStr=uint16  RndMeth=Round
  convert_out : FVT_lib/hal/convert_out  gain=0.125  offset=0
  CAN2_Meter_Ind_VehSpeed : Outport
  wires:
  Data Type Conversion/1 -> CAN2_Meter_Ind_VehSpeed/1
  convert_out/1 -> Data Type Conversion/1
  MeterIndVehSpeed/1 -> convert_out/1

== system halout/HAL_OUT/CAN2/GW2_C10_0_0x1B3/RedWnlmpSta ==
  RedWnlmpSta : Inport
  Data Type Conversion : DataTypeConversion  OutDataTypeStr=uint8  RndMeth=Round
  CAN2_Red_WnlmpSta : Outport
  wires:
  Data Type Conversion/1 -> CAN2_Red_WnlmpSta/1
  RedWnlmpSta/1 -> Data Type Conversion/1

== system halout/HAL_OUT/CAN2/GW2_C10_0_0x1B3/VehSpeed ==
  VehSpeed : Inport
  Data Type Conversion : DataTypeConversion  OutDataTypeStr=uint16  RndMeth=Round
  convert_out : FVT_lib/hal/convert_out  gain=0.125  offset=0
  CAN2_VehSpeed : Outport
  wires:
  Data Type Conversion/1 -> CAN2_VehSpeed/1
  convert_out/1 -> Data Type Conversion/1
  VehSpeed/1 -> convert_out/1

== system halout/HAL_OUT/CAN3/FD3_BCM1_0x216/AllDoorSW ==
  AllDoorSW : Inport
  Data Type Conversion : DataTypeConversion  OutDataTypeStr=uint8  RndMeth=Round
  CAN3_AllDoorSW : Outport
  wires:
  Data Type Conversion/1 -> CAN3_AllDoorSW/1
  AllDoorSW/1 -> Data Type Conversion/1

== system halout/HAL_OUT/CAN3/FD3_BCM1_0x216/AntiTheftSeatFold ==
  AntiTheftSeatFold : Inport
  Data Type Conversion : DataTypeConversion  OutDataTypeStr=uint8  RndMeth=Round
  CAN3_AntiTheftSeatFold : Outport
  wires:
  Data Type Conversion/1 -> CAN3_AntiTheftSeatFold/1
  AntiTheftSeatFold/1 -> Data Type Conversion/1

== system halout/HAL_OUT/CAN3/FD3_BCM1_0x216/AntitheftSta ==
  AntitheftSta : Inport
  Data Type Conversion : DataTypeConversion  OutDataTypeStr=uint8  RndMeth=Round
  CAN3_AntitheftSta : Outport
  wires:
  Data Type Conversion/1 -> CAN3_AntitheftSta/1
  AntitheftSta/1 -> Data Type Conversion/1

== system halout/HAL_OUT/CAN3/FD3_BCM1_0x216/BCMBuzzerReq ==
  BCMBuzzerReq : Inport
  Data Type Conversion : DataTypeConversion  OutDataTypeStr=uint8  RndMeth=Round
  CAN3_BCM_Buzzer_Req : Outport
  wires:
  Data Type Conversion/1 -> CAN3_BCM_Buzzer_Req/1
  BCMBuzzerReq/1 -> Data Type Conversion/1

== system halout/HAL_OUT/CAN3/FD3_BCM1_0x216/BCMDoorLockSta ==
  BCMDoorLockSta : Inport
  Data Type Conversion : DataTypeConversion  OutDataTypeStr=uint8  RndMeth=Round
  CAN3_BCM_DoorLock_Sta : Outport
  wires:
  Data Type Conversion/1 -> CAN3_BCM_DoorLock_Sta/1
  BCMDoorLockSta/1 -> Data Type Conversion/1

== system halout/HAL_OUT/CAN3/FD3_BCM1_0x216/BrakeLamp ==
  BrakeLamp : Inport
  Data Type Conversion : DataTypeConversion  OutDataTypeStr=uint8  RndMeth=Round
  CAN3_BrakeLamp : Outport
  wires:
  Data Type Conversion/1 -> CAN3_BrakeLamp/1
  BrakeLamp/1 -> Data Type Conversion/1

== system halout/HAL_OUT/CAN3/FD3_BCM1_0x216/CTDCtrl ==
  CTDCtrl : Inport
  Data Type Conversion : DataTypeConversion  OutDataTypeStr=uint8  RndMeth=Round
  CAN3_CTDCtrl : Outport
  wires:
  Data Type Conversion/1 -> CAN3_CTDCtrl/1
  CTDCtrl/1 -> Data Type Conversion/1

== system halout/HAL_OUT/CAN3/FD3_BCM1_0x216/CTDLockSW ==
  CTDLockSW : Inport
  Data Type Conversion : DataTypeConversion  OutDataTypeStr=uint8  RndMeth=Round
  CAN3_CTDLockSW : Outport
  wires:
  Data Type Conversion/1 -> CAN3_CTDLockSW/1
  CTDLockSW/1 -> Data Type Conversion/1

== system halout/HAL_OUT/CAN3/FD3_BCM1_0x216/CTDUnlockSW ==
  CTDUnlockSW : Inport
  Data Type Conversion : DataTypeConversion  OutDataTypeStr=uint8  RndMeth=Round
  CAN3_CTDUnlockSW : Outport
  wires:
  Data Type Conversion/1 -> CAN3_CTDUnlockSW/1
  CTDUnlockSW/1 -> Data Type Conversion/1

== system halout/HAL_OUT/CAN3/FD3_BCM1_0x216/CrashDetd ==
  CrashDetd : Inport
  Data Type Conversion : DataTypeConversion  OutDataTypeStr=uint8  RndMeth=Round
  CAN3_CrashDetd : Outport
  wires:
  Data Type Conversion/1 -> CAN3_CrashDetd/1
  CrashDetd/1 -> Data Type Conversion/1

== system halout/HAL_OUT/CAN3/FD3_BCM1_0x216/Dimmer ==
  Dimmer : Inport
  Data Type Conversion : DataTypeConversion  OutDataTypeStr=uint8  RndMeth=Round
  CAN3_Dimmer : Outport
  wires:
  Data Type Conversion/1 -> CAN3_Dimmer/1
  Dimmer/1 -> Data Type Conversion/1

== system halout/HAL_OUT/CAN3/FD3_BCM1_0x216/DimmerEN ==
  DimmerEN : Inport
  Data Type Conversion : DataTypeConversion  OutDataTypeStr=uint8  RndMeth=Round
  CAN3_DimmerEN : Outport
  wires:
  Data Type Conversion/1 -> CAN3_DimmerEN/1
  DimmerEN/1 -> Data Type Conversion/1

== system halout/HAL_OUT/CAN3/FD3_BCM1_0x216/DoorLockIND ==
  DoorLockIND : Inport
  Data Type Conversion : DataTypeConversion  OutDataTypeStr=uint8  RndMeth=Round
  CAN3_DoorLockIND : Outport
  wires:
  Data Type Conversion/1 -> CAN3_DoorLockIND/1
  DoorLockIND/1 -> Data Type Conversion/1

== system halout/HAL_OUT/CAN3/FD3_BCM1_0x216/DrDoorSW ==
  DrDoorSW : Inport
  Data Type Conversion : DataTypeConversion  OutDataTypeStr=uint8  RndMeth=Round
  CAN3_DrDoorSW : Outport
  wires:
  Data Type Conversion/1 -> CAN3_DrDoorSW/1
  DrDoorSW/1 -> Data Type Conversion/1

== system halout/HAL_OUT/CAN3/FD3_BCM1_0x216/FrChargingDoorCtrl ==
  FrChargingDoorCtrl : Inport
  Data Type Conversion : DataTypeConversion  OutDataTypeStr=uint8  RndMeth=Round
  CAN3_Fr_ChargingDoorCtrl : Outport
  wires:
  Data Type Conversion/1 -> CAN3_Fr_ChargingDoorCtrl/1
  FrChargingDoorCtrl/1 -> Data Type Conversion/1

== system halout/HAL_OUT/CAN3/FD3_BCM1_0x216/FrFogLamp ==
  FrFogLamp : Inport
  Data Type Conversion : DataTypeConversion  OutDataTypeStr=uint8  RndMeth=Round
  CAN3_Fr_FogLamp : Outport
  wires:
  Data Type Conversion/1 -> CAN3_Fr_FogLamp/1
  FrFogLamp/1 -> Data Type Conversion/1

== system halout/HAL_OUT/CAN3/FD3_BCM1_0x216/FrWiperH ==
  FrWiperH : Inport
  Data Type Conversion : DataTypeConversion  OutDataTypeStr=uint8  RndMeth=Round
  CAN3_Fr_Wiper_H : Outport
  wires:
  Data Type Conversion/1 -> CAN3_Fr_Wiper_H/1
  FrWiperH/1 -> Data Type Conversion/1

== system halout/HAL_OUT/CAN3/FD3_BCM1_0x216/FrWiperL ==
  FrWiperL : Inport
  Data Type Conversion : DataTypeConversion  OutDataTypeStr=uint8  RndMeth=Round
  CAN3_Fr_Wiper_L : Outport
  wires:
  Data Type Conversion/1 -> CAN3_Fr_Wiper_L/1
  FrWiperL/1 -> Data Type Conversion/1

== system halout/HAL_OUT/CAN3/FD3_BCM1_0x216/HBeam ==
  HBeam : Inport
  Data Type Conversion : DataTypeConversion  OutDataTypeStr=uint8  RndMeth=Round
  CAN3_H_Beam : Outport
  wires:
  Data Type Conversion/1 -> CAN3_H_Beam/1
  HBeam/1 -> Data Type Conversion/1

== system halout/HAL_OUT/CAN3/FD3_BCM1_0x216/HazardSW ==
  HazardSW : Inport
  Data Type Conversion : DataTypeConversion  OutDataTypeStr=uint8  RndMeth=Round
  CAN3_HazardSW : Outport
  wires:
  Data Type Conversion/1 -> CAN3_HazardSW/1
  HazardSW/1 -> Data Type Conversion/1

== system halout/HAL_OUT/CAN3/FD3_BCM1_0x216/HoodSW ==
  HoodSW : Inport
  Data Type Conversion : DataTypeConversion  OutDataTypeStr=uint8  RndMeth=Round
  CAN3_HoodSW : Outport
  wires:
  Data Type Conversion/1 -> CAN3_HoodSW/1
  HoodSW/1 -> Data Type Conversion/1

== system halout/HAL_OUT/CAN3/FD3_BCM1_0x216/HornCtrl ==
  HornCtrl : Inport
  Data Type Conversion : DataTypeConversion  OutDataTypeStr=uint8  RndMeth=Round
  CAN3_HornCtrl : Outport
  wires:
  Data Type Conversion/1 -> CAN3_HornCtrl/1
  HornCtrl/1 -> Data Type Conversion/1

== system halout/HAL_OUT/CAN3/FD3_BCM1_0x216/LAPMWdwEnable ==
  LAPMWdwEnable : Inport
  Data Type Conversion : DataTypeConversion  OutDataTypeStr=uint8  RndMeth=Round
  CAN3_L_APM_WdwEnable : Outport
  wires:
  Data Type Conversion/1 -> CAN3_L_APM_WdwEnable/1
  LAPMWdwEnable/1 -> Data Type Conversion/1

== system halout/HAL_OUT/CAN3/FD3_BCM1_0x216/LBSD ==
  LBSD : Inport
  Data Type Conversion : DataTypeConversion  OutDataTypeStr=uint8  RndMeth=Round
  CAN3_LBSD : Outport
  wires:
  Data Type Conversion/1 -> CAN3_LBSD/1
  LBSD/1 -> Data Type Conversion/1

== system halout/HAL_OUT/CAN3/FD3_BCM1_0x216/LBeam ==
  LBeam : Inport
  Data Type Conversion : DataTypeConversion  OutDataTypeStr=uint8  RndMeth=Round
  CAN3_L_Beam : Outport
  wires:
  Data Type Conversion/1 -> CAN3_L_Beam/1
  LBeam/1 -> Data Type Conversion/1

== system halout/HAL_OUT/CAN3/FD3_BCM1_0x216/LDRL ==
  LDRL : Inport
  Data Type Conversion : DataTypeConversion  OutDataTypeStr=uint8  RndMeth=Round
  CAN3_LDRL : Outport
  wires:
  Data Type Conversion/1 -> CAN3_LDRL/1
  LDRL/1 -> Data Type Conversion/1

== system halout/HAL_OUT/CAN3/FD3_BCM1_0x216/LTurnLP ==
  LTurnLP : Inport
  Data Type Conversion : DataTypeConversion  OutDataTypeStr=uint8  RndMeth=Round
  CAN3_LTurnLP : Outport
  wires:
  Data Type Conversion/1 -> CAN3_LTurnLP/1
  LTurnLP/1 -> Data Type Conversion/1

== system halout/HAL_OUT/CAN3/FD3_BCM1_0x216/LockSetting ==
  LockSetting : Inport
  Data Type Conversion : DataTypeConversion  OutDataTypeStr=uint8  RndMeth=Round
  CAN3_LockSetting : Outport
  wires:
  Data Type Conversion/1 -> CAN3_LockSetting/1
  LockSetting/1 -> Data Type Conversion/1

== system halout/HAL_OUT/CAN3/FD3_BCM1_0x216/MirrorCtrl ==
  MirrorCtrl : Inport
  Data Type Conversion : DataTypeConversion  OutDataTypeStr=uint8  RndMeth=Round
  CAN3_MirrorCtrl : Outport
  wires:
  Data Type Conversion/1 -> CAN3_MirrorCtrl/1
  MirrorCtrl/1 -> Data Type Conversion/1

== system halout/HAL_OUT/CAN3/FD3_BCM1_0x216/MirrorDefog ==
  MirrorDefog : Inport
  Data Type Conversion : DataTypeConversion  OutDataTypeStr=uint8  RndMeth=Round
  CAN3_MirrorDefog : Outport
  wires:
  Data Type Conversion/1 -> CAN3_MirrorDefog/1
  MirrorDefog/1 -> Data Type Conversion/1

== system halout/HAL_OUT/CAN3/FD3_BCM1_0x216/PosLamp ==
  PosLamp : Inport
  Data Type Conversion : DataTypeConversion  OutDataTypeStr=uint8  RndMeth=Round
  CAN3_PosLamp : Outport
  wires:
  Data Type Conversion/1 -> CAN3_PosLamp/1
  PosLamp/1 -> Data Type Conversion/1

== system halout/HAL_OUT/CAN3/FD3_BCM1_0x216/PsDoorSW ==
  PsDoorSW : Inport
  Data Type Conversion : DataTypeConversion  OutDataTypeStr=uint8  RndMeth=Round
  CAN3_PsDoorSW : Outport
  wires:
  Data Type Conversion/1 -> CAN3_PsDoorSW/1
  PsDoorSW/1 -> Data Type Conversion/1

== system halout/HAL_OUT/CAN3/FD3_BCM1_0x216/RBSD ==
  RBSD : Inport
  Data Type Conversion : DataTypeConversion  OutDataTypeStr=uint8  RndMeth=Round
  CAN3_RBSD : Outport
  wires:
  Data Type Conversion/1 -> CAN3_RBSD/1
  RBSD/1 -> Data Type Conversion/1

== system halout/HAL_OUT/CAN3/FD3_BCM1_0x216/RDRL ==
  RDRL : Inport
  Data Type Conversion : DataTypeConversion  OutDataTypeStr=uint8  RndMeth=Round
  CAN3_RDRL : Outport
  wires:
  Data Type Conversion/1 -> CAN3_RDRL/1
  RDRL/1 -> Data Type Conversion/1

== system halout/HAL_OUT/CAN3/FD3_BCM1_0x216/RLDoorSW ==
  RLDoorSW : Inport
  Data Type Conversion : DataTypeConversion  OutDataTypeStr=uint8  RndMeth=Round
  CAN3_RLDoorSW : Outport
  wires:
  Data Type Conversion/1 -> CAN3_RLDoorSW/1
  RLDoorSW/1 -> Data Type Conversion/1

== system halout/HAL_OUT/CAN3/FD3_BCM1_0x216/RRDoorSW ==
  RRDoorSW : Inport
  Data Type Conversion : DataTypeConversion  OutDataTypeStr=uint8  RndMeth=Round
  CAN3_RRDoorSW : Outport
  wires:
  Data Type Conversion/1 -> CAN3_RRDoorSW/1
  RRDoorSW/1 -> Data Type Conversion/1

== system halout/HAL_OUT/CAN3/FD3_BCM1_0x216/RTurnLP ==
  RTurnLP : Inport
  Data Type Conversion : DataTypeConversion  OutDataTypeStr=uint8  RndMeth=Round
  CAN3_RTurnLP : Outport
  wires:
  Data Type Conversion/1 -> CAN3_RTurnLP/1
  RTurnLP/1 -> Data Type Conversion/1

== system halout/HAL_OUT/CAN3/FD3_BCM1_0x216/ReverseLamp ==
  ReverseLamp : Inport
  Data Type Conversion : DataTypeConversion  OutDataTypeStr=uint8  RndMeth=Round
  CAN3_ReverseLamp : Outport
  wires:
  Data Type Conversion/1 -> CAN3_ReverseLamp/1
  ReverseLamp/1 -> Data Type Conversion/1

== system halout/HAL_OUT/CAN3/FD3_BCM1_0x216/RoomLampH ==
  RoomLampH : Inport
  Data Type Conversion : DataTypeConversion  OutDataTypeStr=uint8  RndMeth=Round
  CAN3_RoomLampH : Outport
  wires:
  Data Type Conversion/1 -> CAN3_RoomLampH/1
  RoomLampH/1 -> Data Type Conversion/1

== system halout/HAL_OUT/CAN3/FD3_BCM1_0x216/RoomLampL ==
  RoomLampL : Inport
  Data Type Conversion : DataTypeConversion  OutDataTypeStr=uint8  RndMeth=Round
  CAN3_RoomLampL : Outport
  wires:
  Data Type Conversion/1 -> CAN3_RoomLampL/1
  RoomLampL/1 -> Data Type Conversion/1

== system halout/HAL_OUT/CAN3/FD3_BCM1_0x216/RrChargingDoorCtrl ==
  RrChargingDoorCtrl : Inport
  Data Type Conversion : DataTypeConversion  OutDataTypeStr=uint8  RndMeth=Round
  CAN3_Rr_ChargingDoorCtrl : Outport
  wires:
  Data Type Conversion/1 -> CAN3_Rr_ChargingDoorCtrl/1
  RrChargingDoorCtrl/1 -> Data Type Conversion/1

== system halout/HAL_OUT/CAN3/FD3_BCM1_0x216/RrDefog ==
  RrDefog : Inport
  Data Type Conversion : DataTypeConversion  OutDataTypeStr=uint8  RndMeth=Round
  CAN3_Rr_Defog : Outport
  wires:
  Data Type Conversion/1 -> CAN3_Rr_Defog/1
  RrDefog/1 -> Data Type Conversion/1

== system halout/HAL_OUT/CAN3/FD3_BCM1_0x216/RrFogLamp ==
  RrFogLamp : Inport
  Data Type Conversion : DataTypeConversion  OutDataTypeStr=uint8  RndMeth=Round
  CAN3_Rr_FogLamp : Outport
  wires:
  Data Type Conversion/1 -> CAN3_Rr_FogLamp/1
  RrFogLamp/1 -> Data Type Conversion/1

== system halout/HAL_OUT/CAN3/FD3_BCM1_0x216/RrWiper ==
  RrWiper : Inport
  Data Type Conversion : DataTypeConversion  OutDataTypeStr=uint8  RndMeth=Round
  CAN3_Rr_Wiper : Outport
  wires:
  Data Type Conversion/1 -> CAN3_Rr_Wiper/1
  RrWiper/1 -> Data Type Conversion/1

== system halout/HAL_OUT/CAN3/FD3_BCM1_0x216/TailgateHDSW ==
  TailgateHDSW : Inport
  Data Type Conversion : DataTypeConversion  OutDataTypeStr=uint8  RndMeth=Round
  CAN3_TailgateHDSW : Outport
  wires:
  Data Type Conversion/1 -> CAN3_TailgateHDSW/1
  TailgateHDSW/1 -> Data Type Conversion/1

== system halout/HAL_OUT/CAN3/FD3_BCM1_0x216/TailgateRemote ==
  TailgateRemote : Inport
  Data Type Conversion : DataTypeConversion  OutDataTypeStr=uint8  RndMeth=Round
  CAN3_TailgateRemote : Outport
  wires:
  Data Type Conversion/1 -> CAN3_TailgateRemote/1
  TailgateRemote/1 -> Data Type Conversion/1

== system halout/HAL_OUT/CAN3/FD3_BCM1_0x216/TailgateSW ==
  TailgateSW : Inport
  Data Type Conversion : DataTypeConversion  OutDataTypeStr=uint8  RndMeth=Round
  CAN3_Tailgate_SW : Outport
  wires:
  Data Type Conversion/1 -> CAN3_Tailgate_SW/1
  TailgateSW/1 -> Data Type Conversion/1

== system halout/HAL_OUT/CAN3/FD3_BCM1_0x216/TrunkRel ==
  TrunkRel : Inport
  Data Type Conversion : DataTypeConversion  OutDataTypeStr=uint8  RndMeth=Round
  CAN3_TrunkRel : Outport
  wires:
  Data Type Conversion/1 -> CAN3_TrunkRel/1
  TrunkRel/1 -> Data Type Conversion/1

== system halout/HAL_OUT/CAN3/FD3_BCM1_0x216/WasherCtrl ==
  WasherCtrl : Inport
  Data Type Conversion : DataTypeConversion  OutDataTypeStr=uint8  RndMeth=Round
  CAN3_WasherCtrl : Outport
  wires:
  Data Type Conversion/1 -> CAN3_WasherCtrl/1
  WasherCtrl/1 -> Data Type Conversion/1

== system halout/HAL_OUT/CAN3/FD3_BCM1_0x216/WiperFixMode ==
  WiperFixMode : Inport
  Data Type Conversion : DataTypeConversion  OutDataTypeStr=uint8  RndMeth=Round
  CAN3_WiperFixMode : Outport
  wires:
  Data Type Conversion/1 -> CAN3_WiperFixMode/1
  WiperFixMode/1 -> Data Type Conversion/1
